simulink model "dc_motor"  (R2018a)
settings: Solver=FixedStepAuto  StartTime=0.0  StopTime=inf  FixedStep=SAMPLE_TIME  RelTol=1e-3
values from neighbouring files (symbols this model uses):
  f = 0.00418    [gymmed_test1.mat]    (also in simulation_startup.m = 0; ws_1000_A0B0C0.mat = 0)
  Jm = 0.0104769170021    [gymmed_test1.mat]    (also in simulation_startup.m = 0.046; ws_1000_A0B0C0.mat = 0.0182989442722)
  K = 0.475595317542    [gymmed_test1.mat]    (also in simulation_startup.m = 0.64; ws_1000_A0B0C0.mat = 0.0183378027348)
  L = 2.89835044704e-05    [gymmed_test1.mat]    (also in simulation_startup.m = 0.00059; ws_1000_A0B0C0.mat = 0.0012925545045)
  R = 2.68357079248    [gymmed_test1.mat]    (also in simulation_startup.m = 0.1; ws_1000_A0B0C0.mat = 0.609815109602)
undefined symbols (not defined in the file or in its folder): SAMPLE_TIME
settings Model: Creator=aaronrusso  LastModifiedBy=aaronrusso

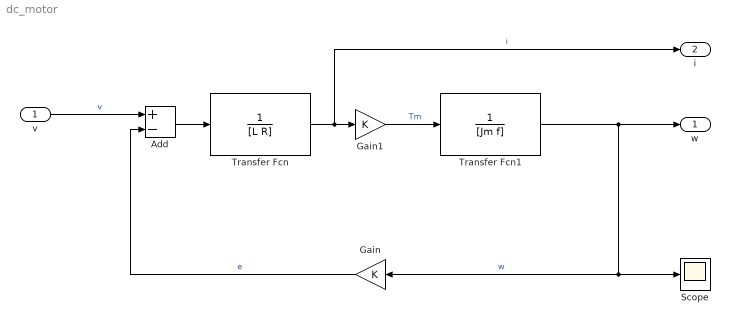
== system dc_motor ==
  v : Inport  SampleTime=SAMPLE_TIME
  Add : Sum  Inputs=+-
  Gain : Gain  Gain=K
  Gain1 : Gain  Gain=K
  Scope : Scope
  Transfer Fcn : TransferFcn  Denominator=[L R]
  Transfer Fcn1 : TransferFcn  Denominator=[Jm f]
  w : Outport  SampleTime=SAMPLE_TIME
  i : Outport  Port=2  SampleTime=SAMPLE_TIME
  wires:
  Transfer Fcn1/1 -> Scope/1, Gain/1, w/1  "w"
  Transfer Fcn/1 -> i/1, Gain1/1  "i"
  Add/1 -> Transfer Fcn/1
  Gain1/1 -> Transfer Fcn1/1  "Tm"
  v/1 -> Add/1  "v"
  Gain/1 -> Add/2  "e"
